simulink library "SPMeTLibrary"  (R2022b)
settings: Solver=VariableStepAuto  StartTime=0.0  StopTime=10.0  RelTol=1e-3
undefined symbols (not defined in the file): model
libraries: simulink x2
settings Model: Creator=ogislason  LastModifiedBy=ogislason

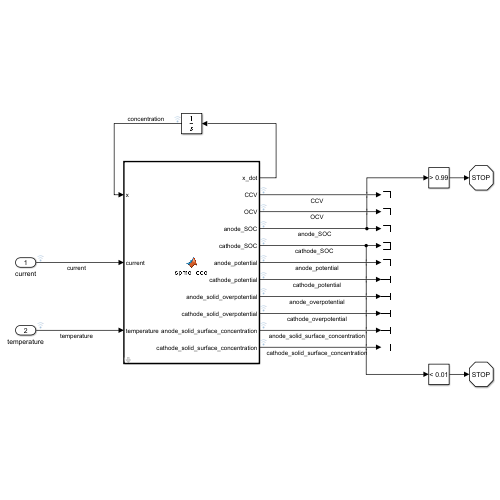
[thumbnail: Simulink's stored preview of the top-level diagram]
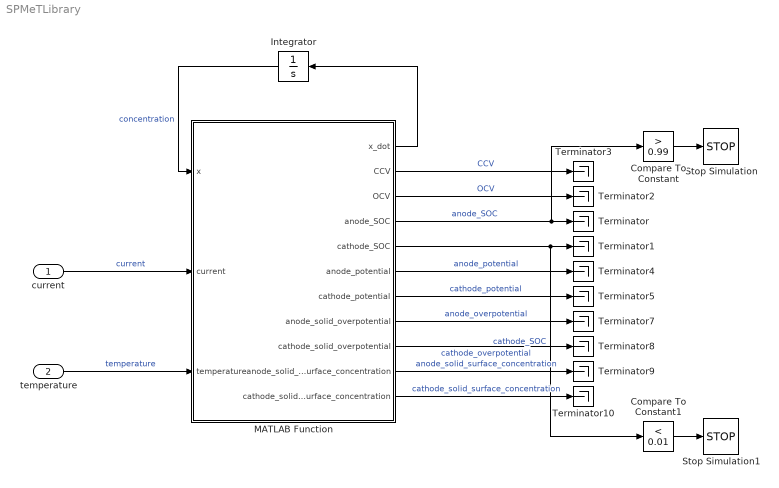
== system SPMeTLibrary ==
  current : Inport
  temperature : Inport  Port=2
  Compare To Constant : simulink/Logic and Bit Operations/Compare To Constant  relop=>  const=0.99  OutDataTypeStr=boolean
  Compare To Constant1 : simulink/Logic and Bit Operations/Compare To Constant  relop=<  const=0.01  OutDataTypeStr=boolean
  Integrator : Integrator  InitialCondition=model.x0
  MATLAB Function : MATLAB Function  TreatAsAtomicUnit=on  mask{cellModel=model}
      mask prompts: cellModel "Cell Model"
  Stop Simulation : Stop
  Stop Simulation1 : Stop
  Terminator{,1..5,7..10} (10 alike) : Terminator
  wires:
  MATLAB Function/8(anode_solid_overpotential) -> Terminator7/1  "anode_overpotential"
  MATLAB Function/10(anode_solid_surface_concentration) -> Terminator9/1  "anode_solid_surface_concentration"
  MATLAB Function/11(cathode_solid_surface_concentration) -> Terminator10/1  "cathode_solid_surface_concentration"
  current/1 -> MATLAB Function/2(current)  "current"
  MATLAB Function/5(cathode_SOC) -> Compare To Constant1/1, Terminator1/1  "cathode_SOC"
  Compare To Constant/1 -> Stop Simulation/1
  MATLAB Function/2(CCV) -> Terminator3/1  "CCV"
  Compare To Constant1/1 -> Stop Simulation1/1
  MATLAB Function/7(cathode_potential) -> Terminator5/1  "cathode_potential"
  MATLAB Function/4(anode_SOC) -> Compare To Constant/1, Terminator/1  "anode_SOC"
  MATLAB Function/6(anode_potential) -> Terminator4/1  "anode_potential"
  temperature/1 -> MATLAB Function/3(temperature)  "temperature"
  MATLAB Function/1(x_dot) -> Integrator/1
  Integrator/1 -> MATLAB Function/1(x)  "concentration"
  MATLAB Function/3(OCV) -> Terminator2/1  "OCV"
  MATLAB Function/9(cathode_solid_overpotential) -> Terminator8/1  "cathode_overpotential"

== matlab function SPMeTLibrary/MATLAB Function ==
  data: model parameter; x_dot output size=height(model.x0); x input size=height(model.x0); current input size=1; temperature input size=1; CCV output size=1; OCV output size=1; anode_SOC output size=1; cathode_SOC output size=1; anode_potential output; cathode_potential output; anode_solid_overpotential output; cathode_solid_overpotential output; anode_solid_surface_concentration output; cathode_solid_surface_concentration output
function [x_dot,CCV,OCV,anode_SOC,cathode_SOC,anode_potential,cathode_potential,...
    anode_solid_overpotential,cathode_solid_overpotential,...
    anode_solid_surface_concentration,cathode_solid_surface_concentration]  = spme_ode(model,x,current,temperature)
temperature = temperature+273.15;
%% Shorthand
anode = model.anode;
cathode = model.cathode;
% Parse states
anode_solid_concentration   = x(1:(model.discretization.radial_divisions-1));
cathode_solid_concentration = x(model.discretization.radial_divisions : 2*(model.discretization.radial_divisions-1));
electrolyte_concentration   = x(2*model.discretization.radial_divisions-1 : 2*model.discretization.radial_divisions-1+model.discretization.Nx-4);
delta_sei = x(end);

%% Pre-calculations with current states

%%% MOLAR FLUXES
% Compute total molar flux
anode_total_molar_flux =  current/(F*  anode.specific_interfacial_area*model.electrode_area*  anode.electrode_thickness);
cathode_total_molar_flux = -current/(F*cathode.specific_interfacial_area*model.electrode_area*cathode.electrode_thickness);

%%% SOLID PHASE DYNAMICS
% Solid phase diffusivity temperature dependence
anode_diffusion_coefficient   = anode.diffusion_coefficient * exp(anode.diffusion_activation_energy/R*(1/model.nominal_temperature - 1/temperature));
cathode_diffusion_coefficient = cathode.diffusion_coefficient * exp(cathode.diffusion_activation_energy/R*(1/model.nominal_temperature - 1/temperature));

% Construct (A,B) matrices for solid-phase Li diffusion
model = initialize_solid_phase_matrices(model,anode_diffusion_coefficient,cathode_diffusion_coefficient);
% Compute surface concentrations
anode_solid_surface_concentration = model.solid_phase_matrices.C_n*anode_solid_concentration + model.solid_phase_matrices.D_n*anode_total_molar_flux;
cathode_solid_surface_concentration = model.solid_phase_matrices.C_p*cathode_solid_concentration + model.solid_phase_matrices.D_p*cathode_total_molar_flux;
% Remark: I am cheating slightly here. jn_tot should be jn, but doing so
% imposes an algebraic equation. This forms a DAE. I am going to
% approximate jn by jn_tot, which should be ok, since jn and jn_tot have a
% error on the order of 0.001%


%%% ELECTROLYTE PHASE DYNAMICS
% Compute electrolyte Boundary Conditions
electrolyte_concentration_boundary_conditions = model.electrolyte_matrices.C * electrolyte_concentration;

ce0n = electrolyte_concentration_boundary_conditions(1);
cens = electrolyte_concentration_boundary_conditions(2);
cesp = electrolyte_concentration_boundary_conditions(3);
ce0p = electrolyte_concentration_boundary_conditions(4);

% Separate and aggregate electrolyte concentration
anode_electrolyte_concentration = electrolyte_concentration(1:(model.discretization.Nxn-1));
separator_electrolyte_concentration = electrolyte_concentration((model.discretization.Nxn-1)+1:(model.discretization.Nxn-1)+(model.discretization.Nxs-1));
cathode_electrolyte_concentration = electrolyte_concentration((model.discretization.Nxn-1)+model.discretization.Nxs : end);
electrolyte_concentrations = [ce0n; anode_electrolyte_concentration; cens; separator_electrolyte_concentration; cesp; cathode_electrolyte_concentration; ce0p];

% Average electrolyte concentrations
mean_electrolyte_concentration_anode = mean(electrolyte_concentrations(1:model.discretization.Nxn+1,:));
mean_electrolyte_concentration_separator = mean(electrolyte_concentrations((model.discretization.Nxn+1):(model.discretization.Nxn+model.discretization.Nxs+1),:));
mean_electrolyte_concentration_cathode = mean(electrolyte_concentrations((model.discretization.Nxn+model.discretization.Nxs+1):(model.discretization.Nxn+model.discretization.Nxs+model.discretization.Nxp+1),:));

% Overpotentials due to electrolyte subsystem
nominal_electrolyte_conductivity_anode = electrolyteCond(mean_electrolyte_concentration_anode);
nominal_electrolyte_conductivity_separator = electrolyteCond(mean_electrolyte_concentration_separator);
nominal_electrolyte_conductivity_cathode = electrolyteCond(mean_electrolyte_concentration_cathode);

% Adjustment for Arrhenius temperature dependence
temperature_scaling_factor = exp(model.electrolyte.conductivity_activation_energy/R*(1/model.nominal_temperature - 1/temperature));
anode_electrolyte_conductivity = nominal_electrolyte_conductivity_anode * temperature_scaling_factor;
separator_electrolyte_conductivity = nominal_electrolyte_conductivity_separator * temperature_scaling_factor;
cathode_electrolyte_conductivity = nominal_electrolyte_conductivity_cathode * temperature_scaling_factor;

% Bruggeman relationships
effective_anode_electrolyte_conductivity = anode_electrolyte_conductivity * anode.volume_fraction_electrolyte.^(model.bruggemann_porosity);
effective_separator_electrolyte_conductivity = separator_electrolyte_conductivity * model.separator.volume_fraction_electrolyte.^(model.bruggemann_porosity);
effective_cathode_electrolyte_conductivity = cathode_electrolyte_conductivity * cathode.volume_fraction_electrolyte.^(model.bruggemann_porosity);

% Activity coefficient
dfca_n = electrolyteAct(model,mean_electrolyte_concentration_anode,temperature);
dfca_s = electrolyteAct(model,mean_electrolyte_concentration_separator,temperature);
dfca_p = electrolyteAct(model,mean_electrolyte_concentration_cathode,temperature);

% Kinetic reaction rate, adjusted for Arrhenius temperature dependence
anode_reaction_rate   =   anode.reaction_rate * exp(  anode.intercalation_activation_energy/R*(1/model.nominal_temperature - 1/temperature));
cathode_reaction_rate = cathode.reaction_rate * exp(cathode.intercalation_activation_energy/R*(1/model.nominal_temperature - 1/temperature));

% Stochiometric Concentration Ratio
theta_n = anode_solid_surface_concentration / anode.maximum_concentration;
theta_p = cathode_solid_surface_concentration / cathode.maximum_concentration;

% Exchange current density
mean_electrolyte_concentrations = [mean_electrolyte_concentration_anode; mean_electrolyte_concentration_separator; mean_electrolyte_concentration_cathode];
[i_0n,i_0p] = exch_cur_dens(model,cathode_reaction_rate,anode_reaction_rate,anode_solid_surface_concentration,cathode_solid_surface_concentration,mean_electrolyte_concentrations);

%% Voltage output
% Equilibrium Potential
anode_reference_potential = refPotentialAnode(theta_n);
cathode_reference_potential = refPotentialCathode(theta_p);

% Overpotentials
RTaF=(R*temperature)/(model.charge_transfer_coefficient*F);
anode_solid_overpotential   = RTaF * asinh( current / (2*anode.specific_interfacial_area  *model.electrode_area*anode.electrode_thickness  *i_0n(1)));
cathode_solid_overpotential = RTaF * asinh(-current / (2*cathode.specific_interfacial_area*model.electrode_area*cathode.electrode_thickness*i_0p(end)));

% Total resistance (film + growing SEI layer)
anode_resistivity = anode.sei_resistivity + delta_sei/model.side_reaction_product.conductivity;
anode_resistance = anode_resistivity/(anode.specific_interfacial_area*anode.electrode_thickness*model.electrode_area);
cathode_resistivity = 0;
cathode_resistance = cathode_resistivity/(cathode.specific_interfacial_area*cathode.electrode_thickness*model.electrode_area);
%Solid phase voltage drop
anode_solid_IR = anode_resistance*current;
cathode_solid_IR= cathode_resistance*current;
% Overpotential due to electrolyte resistance
anode_electrolyte_IR = anode.electrode_thickness/(2*effective_anode_electrolyte_conductivity)*current;
separator_electrolyte_IR = 2*model.separator.thickness/(2*effective_separator_electrolyte_conductivity)*current;
cathode_electrolyte_IR = cathode.electrode_thickness/(2*effective_cathode_electrolyte_conductivity)*current;

% Overpotential due to electrolyte polarization
anode_electrolyte_overpotential =  (2*R*temperature)/(F) * (1-model.transference_number)* (1+dfca_n) * (log(cens) - log(ce0n));
separator_electrolyte_overpotential = (2*R*temperature)/(F) * (1-model.transference_number) * (1+dfca_s) * (log(cesp) - log(cens));
cathode_electrolyte_overpotential = (2*R*temperature)/(F) * (1-model.transference_number) * (1+dfca_p) * (log(ce0p) - log(cesp));

anode_potential   = anode_reference_potential + anode_solid_overpotential + anode_solid_IR - anode_electrolyte_overpotential - anode_electrolyte_IR;
cathode_potential = cathode_reference_potential + cathode_solid_overpotential  - cathode_solid_IR  + cathode_electrolyte_overpotential + cathode_electrolyte_IR;
separator_potential = separator_electrolyte_IR + separator_electrolyte_overpotential;

CCV = cathode_potential - anode_potential + separator_potential;

%% Aging Dynamics

%   SEI Layer Growth model
%   Eqns Adopted from Ramadass et al (2004) [Univ of South Carolina]
%   "Development of First Principles Capacity Fade Model for Li-Ion Cells"
%   DOI: 10.1149/1.1634273
%   NOTE1: This model has NOT been validated experimentally by eCAL
%   NOTE2: We assume this submodel only applies to anode

% Difference btw solid and electrolyte overpotential [V]
phi_se = anode_solid_overpotential + anode_reference_potential + F*anode_resistivity*anode_total_molar_flux;

% Side rxn overpotential [V]
eta_s = phi_se - model.side_reaction_product.reference_potential - F*anode_resistivity * anode_total_molar_flux;

% Molar flux of side rxn [mol/s-m^2]
j_s = -model.side_reaction_product.exchange_current_density/...
    F * exp((-model.charge_transfer_coefficient*F)/(R*temperature)*eta_s);

% SEI layer growth model [m/s]
delta_sei_dot = -model.side_reaction_product.molecular_weight/...
    (model.side_reaction_product.mass_density) * j_s;

% Molar flux of intercalation
jn = (abs(anode_total_molar_flux) - abs(j_s)) * sign(anode_total_molar_flux);
jp = cathode_total_molar_flux;

%% Solid Phase Dynamics
% ODE for c_s
anode_solid_concentration_dot = model.solid_phase_matrices.A_n*anode_solid_concentration + model.solid_phase_matrices.B_n*jn;
cathode_solid_concentration_dot = model.solid_phase_matrices.A_p*cathode_solid_concentration + model.solid_phase_matrices.B_p*jp;

%% Electrolyte Dynamics

% Compute Electrolyte Diffusion Coefficient and Derivative
[D_en0,dD_en0] = electrolyte_diffusion_coefficient(anode_electrolyte_concentration);
[D_es0,dD_es0] = electrolyte_diffusion_coefficient(separator_electrolyte_concentration);
[D_ep0,dD_ep0] = electrolyte_diffusion_coefficient(cathode_electrolyte_concentration);

% Adjustment for Arrhenius temperature dependence
Arrh_De = exp(model.electrolyte.diffusion_activation_energy/R*(1/model.nominal_temperature - 1/temperature));
D_en = D_en0 * Arrh_De;
D_es = D_es0 * Arrh_De;
D_ep = D_ep0 * Arrh_De;
dD_en = dD_en0 * Arrh_De;
dD_es = dD_es0 * Arrh_De;
dD_ep = dD_ep0 * Arrh_De;

% Apply BRUGGEMAN RELATION
D_en_eff = D_en .* anode.volume_fraction_electrolyte.^(model.bruggemann_porosity-1);
dD_en_eff = dD_en .* anode.volume_fraction_electrolyte.^(model.bruggemann_porosity-1);

D_es_eff = D_es .* model.separator.volume_fraction_electrolyte.^(model.bruggemann_porosity-1);
dD_es_eff = dD_es .* model.separator.volume_fraction_electrolyte.^(model.bruggemann_porosity-1);

D_ep_eff = D_ep .* cathode.volume_fraction_electrolyte.^(model.bruggemann_porosity-1);
dD_ep_eff = dD_ep .* cathode.volume_fraction_electrolyte.^(model.bruggemann_porosity-1);

% Compute derivative

anode_electrolyte_concentration_dot = dD_en_eff.*(model.electrolyte_matrices.M1n*anode_electrolyte_concentration + model.electrolyte_matrices.M2n*electrolyte_concentration_boundary_conditions(1:2)).^2 ...
    + D_en_eff.*(model.electrolyte_matrices.M3n*anode_electrolyte_concentration + model.electrolyte_matrices.M4n*electrolyte_concentration_boundary_conditions(1:2)) + diag(model.electrolyte_matrices.M5n)*jn;

separator_electrolyte_concentration_dot = dD_es_eff.*(model.electrolyte_matrices.M1s*separator_electrolyte_concentration + model.electrolyte_matrices.M2s*electrolyte_concentration_boundary_conditions(2:3)).^2 ...
    + D_es_eff.*(model.electrolyte_matrices.M3s*separator_electrolyte_concentration + model.electrolyte_matrices.M4s*electrolyte_concentration_boundary_conditions(2:3));

cathode_electrolyte_concentration_dot = dD_ep_eff.*(model.electrolyte_matrices.M1p*cathode_electrolyte_concentration + model.electrolyte_matrices.M2p*electrolyte_concentration_boundary_conditions(3:4)).^2 ...
    + D_ep_eff.*(model.electrolyte_matrices.M3p*cathode_electrolyte_concentration + model.electrolyte_matrices.M4p*electrolyte_concentration_boundary_conditions(3:4)) + diag(model.electrolyte_matrices.M5p)*jp;

% Assemble c_e_dot
electrolyte_concentration_dot = [anode_electrolyte_concentration_dot; separator_electrolyte_concentration_dot; cathode_electrolyte_concentration_dot];

%% Thermal Dynamics

% State-of-Charge (Bulk)
r_vec = (0:model.discretization.delta_r_n:1)';
c_n = [anode_solid_concentration(1); anode_solid_concentration; anode_solid_surface_concentration];
c_p = [cathode_solid_concentration(1); cathode_solid_concentration; cathode_solid_surface_concentration];
anode_SOC = 3/anode.maximum_concentration * trapz(r_vec,r_vec.^2.*c_n);
cathode_SOC = 3/cathode.maximum_concentration * trapz(r_vec,r_vec.^2.*c_p);

% Equilibrium potentials
[anode_OCV] = refPotentialAnode(anode_SOC);
[cathode_OCV] = refPotentialCathode(cathode_SOC);
OCV = cathode_OCV - anode_OCV;

%% Concatenate time derivatives
x_dot = [anode_solid_concentration_dot; cathode_solid_concentration_dot; electrolyte_concentration_dot; delta_sei_dot];

end
